simulink model "slxcases_R2013b"  (R2013b)
settings: Solver=ode45  SolverMode=SingleTasking  StartTime=0.0  StopTime=10.0  RelTol=1e-3
model workspace (MAT data in the model file):
  cfg.mode = 'fast'
  cfg.gain = 2
  flag = 1
  grid = [1  2  3; 4  5  6]
  inner = 7
  label = 'hello'
  names = {'alpha', 'beta'}
  span = 3
  tau = 0.25
undefined symbols (not defined in the file or in its folder): Ki, Kp
settings Model: CovMetricSettings=d  CovHtmlReporting=off  covSaveCumulativeToWorkspaceVar=off  CovSaveSingleToWorkspaceVar=off  CovExternalEMLEnable=on  Creator=weiwang  LastModifiedBy=weiwang
settings DataIOCC: LimitDataPoints=off  SaveFormat=StructureWithTime  ReturnWorkspaceOutputs=on
settings DebuggingCC: UnderspecifiedInitializationDetection=Simplified  MergeDetectMultiDrivingBlocksExec=error  SolverPrmCheckMsg=none  UnconnectedInputMsg=none  UnconnectedOutputMsg=none  UnconnectedLineMsg=none  SFUnexpectedBacktrackingDiag=error  SFNoUnconditionalDefaultTransitionDiag=error
settings HardwareCC: ProdBitPerPointer=64  ProdLargestAtomicFloat=Float  ProdIntDivRoundTo=Zero  ProdEndianess=LittleEndian  ProdHWDeviceType=Specified
settings ModelReferenceCC: UpdateModelReferenceTargets=IfOutOfDate  PropagateSignalLabelsOutOfModel=on
settings SFSimCC: SimUseLocalCustomCode=on
settings RTWCC: RTWUseLocalCustomCode=on
settings GRTTargetCC: CodeReplacementLibrary=C99 (ISO)

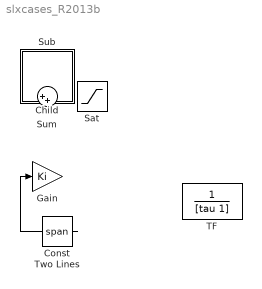
== system slxcases_R2013b ==
  Child : ModelReference  ModelNameDialog=slx_child  ModelReferenceVersion=1.1
  Const : Constant  Value=Kp
  Gain : Gain  Gain=Ki
  Sat : Saturate  UpperLimit=Inf  LowerLimit=-Inf
  Sub : Subsystem
  Sum : Sum  Inputs=|++
  TF : TransferFcn  Denominator=[tau 1]
  Two Lines : Constant  Value=span
  wires:
  Const/1 -> Gain/1

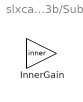
== system slxcases_R2013b/Sub ==
  InnerGain : Gain  Gain=inner
